simulink model "ccmodel"  (R2021b)
settings: Solver=VariableStepAuto  StartTime=0.0  StopTime=120  RelTol=1e-3
undefined symbols (not defined in the file): b, m
settings Model: Creator=feyzi  LastModifiedBy=feyzi

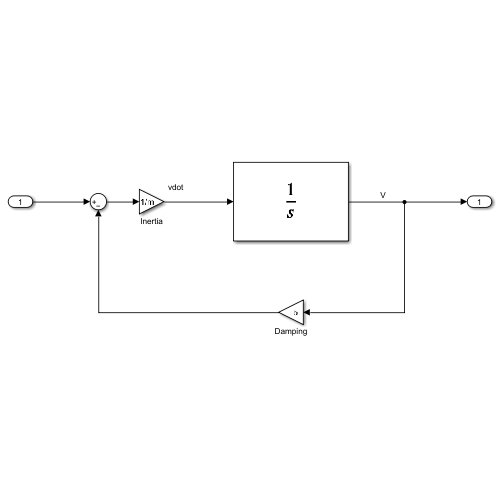
[thumbnail: Simulink's stored preview of the top-level diagram]
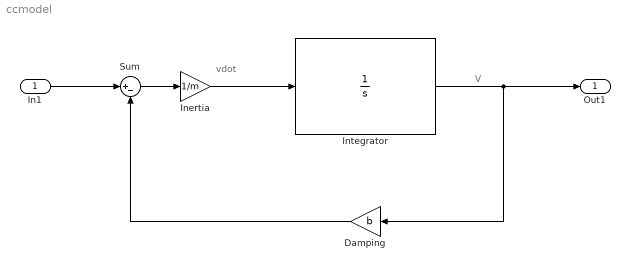
== system ccmodel ==
  note: V
  note: vdot
  In1 : Inport
  Damping : Gain  Gain=b
  Inertia : Gain  Gain=1/m
  Integrator : Integrator  ContinuousStateAttributes="\"Integrator\""
  Sum : Sum  Inputs=|+-
  Out1 : Outport
  wires:
  Integrator/1 -> Out1/1, Damping/1
  Inertia/1 -> Integrator/1
  Damping/1 -> Sum/2
  Sum/1 -> Inertia/1
  In1/1 -> Sum/1
